simulink model "Cart_Pendulum_Linearised_b_n9558292"  (R2018a)
settings: Solver=VariableStepAuto  StartTime=0.0  StopTime=10.0  RelTol=1e-3
values from neighbouring files (symbols this model uses):
  g = 9.81    [MainFile_Linearised_a_n9558292.m]    (also in MainFile_Linearised_b_n9558292.m; MainFile_n9558292.m)
  l = 0.2    [MainFile_Linearised_a_n9558292.m]    (also in MainFile_Linearised_b_n9558292.m; MainFile_n9558292.m)
  m = 0.15    [MainFile_Linearised_a_n9558292.m]    (also in MainFile_Linearised_b_n9558292.m; MainFile_n9558292.m)
  Mc = 0.4    [MainFile_Linearised_a_n9558292.m]    (also in MainFile_Linearised_b_n9558292.m; MainFile_n9558292.m)
  stepfb_tilde = 0.1    [MainFile_Linearised_b_n9558292.m]
  stepib_tilde = 0    [MainFile_Linearised_b_n9558292.m]
  steptb_tilde = 1    [MainFile_Linearised_b_n9558292.m]
  x10b_tilde = 0    [MainFile_Linearised_b_n9558292.m]
  x20b_tilde = pi    (= 3.14159265359)    [MainFile_Linearised_b_n9558292.m]
  x30b_tilde = 0    [MainFile_Linearised_b_n9558292.m]
  x40b_tilde = 0    [MainFile_Linearised_b_n9558292.m]
settings Model: Creator=haidarobeid  LastModifiedBy=haidarobeid
settings DataIOCC: SaveFormat=Array  TimeSaveName=toutb_tilde

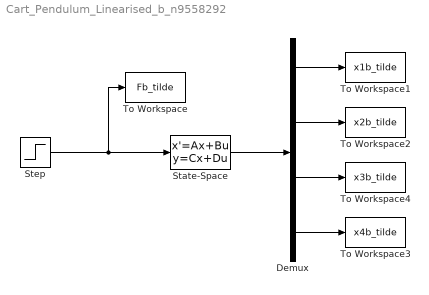
== system Cart_Pendulum_Linearised_b_n9558292 ==
  Demux : Demux
  State-Space : StateSpace  A=[0,0,1,0;0,0,0,1;0,-m*g/Mc,0,0;0,-g*(Mc+m)/(l*Mc),0,0]  B=[0;0;1/Mc;1/(l*Mc)]  C=eye(4)  D=[0; 0; 0 ;0]  InitialCondition=[x10b_tilde;x20b_tilde;x30b_tilde;x40b_tilde]
  Step : Step  Time=steptb_tilde  Before=stepib_tilde  After=stepfb_tilde  SampleTime=0
  To Workspace : ToWorkspace  VariableName=Fb_tilde  SampleTime=-1
  To Workspace1 : ToWorkspace  VariableName=x1b_tilde  SampleTime=-1
  To Workspace2 : ToWorkspace  VariableName=x2b_tilde  SampleTime=-1
  To Workspace3 : ToWorkspace  VariableName=x4b_tilde  SampleTime=-1
  To Workspace4 : ToWorkspace  VariableName=x3b_tilde  SampleTime=-1
  wires:
  Demux/1 -> To Workspace1/1
  Step/1 -> To Workspace/1, State-Space/1
  Demux/4 -> To Workspace3/1
  Demux/2 -> To Workspace2/1
  State-Space/1 -> Demux/1
  Demux/3 -> To Workspace4/1
